simulink model "N2 blowdown"  (R2020a)
settings: Solver=VariableStepAuto  StartTime=0.0  StopTime=10.0  RelTol=1e-3
settings Model: Creator=parthmahendru  LastModifiedBy=parthmahendru

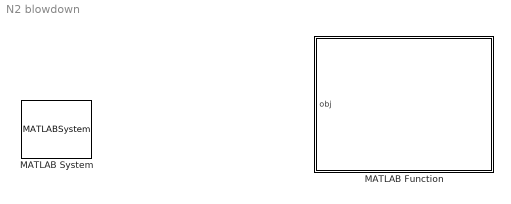
== system N2 blowdown ==
  MATLAB Function : MATLAB Function  TreatAsAtomicUnit=on
  MATLAB System : MATLABSystem  System=shumshing  Gain=1.5  Bias=0.1  SimulateUsing=Code generation
      mask Type: shumshing
      mask Display:
      | disp('shumshing');
      | port_label('input',1,'u');
      | port_label('output',1,'y');

== matlab function N2 blowdown/MATLAB Function ==
  data: obj input
        function          OX_constantPressureBlowdown(obj)

            mDot             = obj.input.design.mDotox;
            T                = obj.input.(obj.inputTag).Tinit;
            
            V                = obj.tank.v;
            mTank            = obj.tank.m;
            P                = IC.P;
            n                = IC.n;
            Cd               = obj.input.design.injCd;
            Pe               = Pcc  * cnv;
            nPres            = m(1, 1)/MW;
            model            = fluidModel;

            in                  = obj.findAinj(in);

            for i = 2 : obj.input.sim.numpt

                out             = blowdownCharacteristics(in);
                dP              = P(i - 1, 1) - out.P;

                while (dP > obj.input.settings.dPtol)

                    nPres        = nPres  + obj.input.settings.npr_inc;
                    out             = blowdownCharacteristics(in);
                    dP              = P(i - 1, 1)   - out.P;
                end

                n(i, :)      = n(i-1, :) + out.dn * obj.input.sim.dt;
                T(i, :)      = T(i-1, 1) + out.dT * obj.input.sim.dt;
                mdot(i, 1)   = out.mDot;
                P(i, :)      = [out.P, out.P];
                
                n(i, 1)      = nPres;

                T                        = T(i, 1);
                n                        = n(i, :);
                P                        = P(i, 1);
            end

            m        = n * MW;
            m        = n * MW;
        end
